simulink model "sinvel"  (R2017a)
settings: Solver=FixedStepAuto  StartTime=0.0  StopTime=inf  RelTol=1e-3  EnableMultiTasking=on
undefined symbols (not defined in the file): Angular, Linear
libraries: robotlib x2
settings Model: Creator=ece446  LastModifiedBy=ece446
settings OptimizationCC: LifeSpan=Inf  MaxStackSize=64
settings DebuggingCC: SFUnexpectedBacktrackingDiag=warning  SFNoUnconditionalDefaultTransitionDiag=warning  SFExecutionAtInitializationDiag=none
settings HardwareCC: ProdBitPerPointer=32  ProdBitPerSizeT=32  ProdBitPerPtrDiffT=32  ProdLargestAtomicFloat=None  ProdIntDivRoundTo=Undefined  ProdEndianess=Unspecified  ProdWordSize=32  ProdHWDeviceType=Generic->Unspecified (assume 32-bit Generic)  UseEmbeddedCoderFeatures=off
settings RTWCC: SystemTargetFile=ert.tlc  HardwareBoard=Robot Operating System (ROS)  TLCOptions=-aInlineSetEventsForThisBaseRateFcn=TLC_FALSE -aSuppressMultiTaskScheduler=TLC_FALSE -aRateBasedStepFcn=0  TemplateMakefile=ert_default_tmf  Description=Embedded Coder  GenerateReport=on  Toolchain=Catkin  LaunchReport=on  TargetLang=C++
settings CodeAppCC: ForceParamTrailComments=on  OperatorAnnotations=on  MATLABSourceComments=on
settings ERTTargetCC: MultiwordLength=2048  ERTCustomFileBanners=off  SupportContinuousTime=on  SupportNonInlinedSFcns=on  RemoveResetFunc=off  ModelStepFunctionPrototypeControlCompliant=off
settings ConfigComp: CovMetricSettings=dw  CovHtmlReporting=on  CovSaveCumulativeToWorkspaceVar=on  CovSaveSingleToWorkspaceVar=on  CovExternalEMLEnable=off

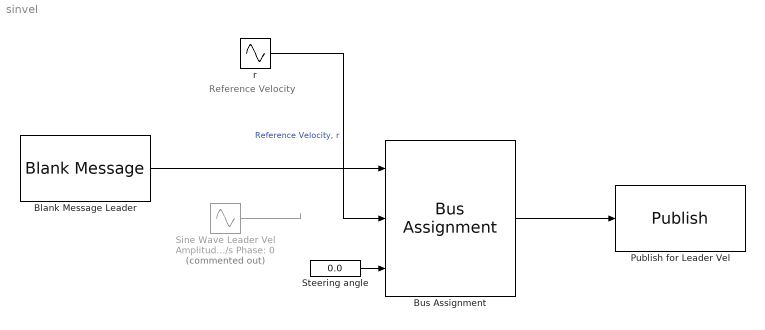
== system sinvel ==
  note: Reference Velocity
  Blank Message Leader : robotlib/Blank Message  SourceLibraryInfo=This block requires Robotics System Toolbox  messageType=geometry_msgs/Twist  SampleTime=inf
      settings: SourceProductBaseCode=RO
  Bus Assignment : BusAssignment  AssignedSignals=Linear.X,Angular.Z
  Publish for Leader Vel : robotlib/Publish  SourceLibraryInfo=This block requires Robotics System Toolbox  topicSource=Select from ROS network  topic=/azcar_sim/cmd_vel  messageType=geometry_msgs/Twist  messageQueueLength=1
      settings: SourceProductBaseCode=RO
  "Sine Wave Leader Vel Amplitude: 4 Bias: 3 Frequency: 5/2*pi rad/s Phase: 0 " : Sin  Commented=on  Amplitude=4.0  Bias=3  Frequency=0.7958  SampleTime=0
  Steering angle : Constant  Value=0.0
  r : Sin  Amplitude=2  Bias=2  Frequency=0.25  Phase=0.12  SampleTime=0
  wires:
  Blank Message Leader/1 -> Bus Assignment/1
  Bus Assignment/1 -> Publish for Leader Vel/1
  "Sine Wave Leader Vel Amplitude: 4 Bias: 3 Frequency: 5/2*pi rad/s Phase: 0 "/1 -> ?
  Steering angle/1 -> Bus Assignment/3
  r/1 -> Bus Assignment/2  "Reference Velocity, r"
